simulink model "PAlab3_5_1"  (R2025a)
settings: Solver=VariableStepAuto  StartTime=0.0  StopTime=10.0  RelTol=1e-3
settings Model: Creator=mieszko  LastModifiedBy=Acer

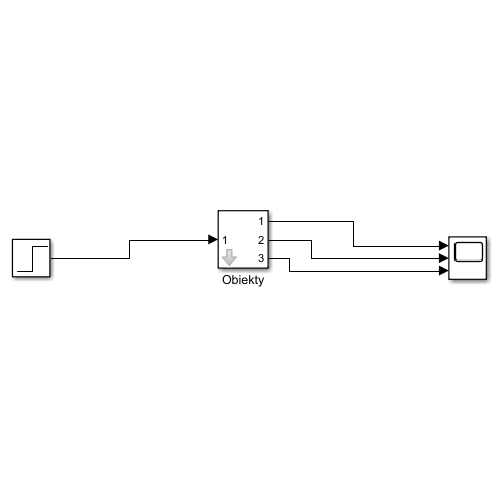
[thumbnail: Simulink's stored preview of the top-level diagram]
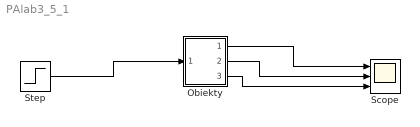
== system PAlab3_5_1 ==
  Obiekty : Subsystem  mask{k1=5, k2=2, k3=3}
  Scope : Scope  NumInputPorts=3
      settings: ActiveDisplayYMinimum=-12.498457375854635  ActiveDisplayYMaximum=112.48611638269175
  Step : Step  SampleTime=0
  wires:
  Step/1 -> Obiekty/1(In1)
  Obiekty/1(Out1) -> Scope/1
  Obiekty/2(Out2) -> Scope/2
  Obiekty/3(Out3) -> Scope/3

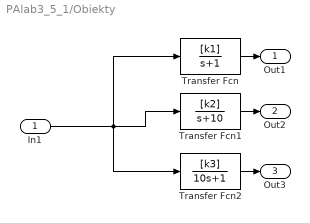
== system PAlab3_5_1/Obiekty ==
  In1 : Inport
  Transfer Fcn : TransferFcn  Numerator=[k1]  Denominator=[1 1]
  Transfer Fcn1 : TransferFcn  Numerator=[k2]  Denominator=[1 10]
  Transfer Fcn2 : TransferFcn  Numerator=[k3]  Denominator=[10 1]
  Out1 : Outport
  Out2 : Outport  Port=2
  Out3 : Outport  Port=3
  wires:
  Transfer Fcn/1 -> Out1/1
  Transfer Fcn1/1 -> Out2/1
  Transfer Fcn2/1 -> Out3/1
  In1/1 -> Transfer Fcn1/1, Transfer Fcn/1, Transfer Fcn2/1
